simulink model "practica"  (R2014a)
settings: Solver=ode45  StartTime=0.0  StopTime=10.0  RelTol=1e-3
values from neighbouring files (symbols this model uses):
  C1 = 1e-6    (= 1e-06)    [practica8.m]
  C2 = 1e-6    (= 1e-06)    [practica8.m]
  f = 40    [practica8.m]
  R1 = 4.7e3    (= 4700)    [practica8.m]
  R2 = 3.6e3    (= 3600)    [practica8.m]
  Vm = 10    [practica8.m]
settings Model: Creator=Diana  LastModifiedBy=Diana

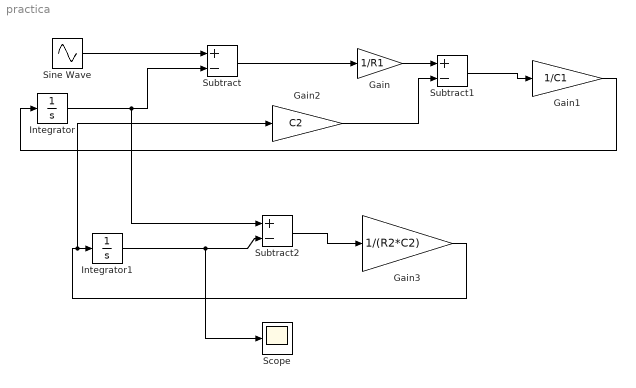
== system practica ==
  Gain : Gain  Gain=1/R1
  Gain1 : Gain  Gain=1/C1
  Gain2 : Gain  Gain=C2
  Gain3 : Gain  Gain=1/(R2*C2)
  Integrator : Integrator
  Integrator1 : Integrator
  Scope : Scope
  Sine Wave : Sin  Amplitude=Vm  Frequency=2*pi*f  SampleTime=0
  Subtract : Sum  Inputs=+-
  Subtract1 : Sum  Inputs=+-
  Subtract2 : Sum  Inputs=+-
  wires:
  Sine Wave/1 -> Subtract/1
  Subtract/1 -> Gain/1
  Gain/1 -> Subtract1/1
  Subtract1/1 -> Gain1/1
  Gain1/1 -> Integrator/1
  Integrator/1 -> Subtract2/1, Subtract/2
  Integrator1/1 -> Scope/1, Subtract2/2
  Gain2/1 -> Subtract1/2
  Subtract2/1 -> Gain3/1
  Gain3/1 -> Gain2/1, Integrator1/1
